simulink library "DYN_SRP"  (Simulink 8.8)
settings: Solver=ode45  StartTime=0.0  StopTime=10.0  RelTol=1e-3  EnableMultiTasking=on
undefined symbols (not defined in the file): CONSTANTS_par, DYN_SC_par
libraries: LIB_ROT x3, LIB_DYN x1, LIB_ENV x1
settings Model: Creator=alger  LastModifiedBy=alger

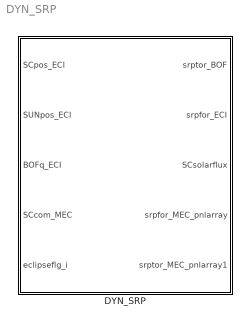
== system DYN_SRP ==
  DYN_SRP : Subsystem

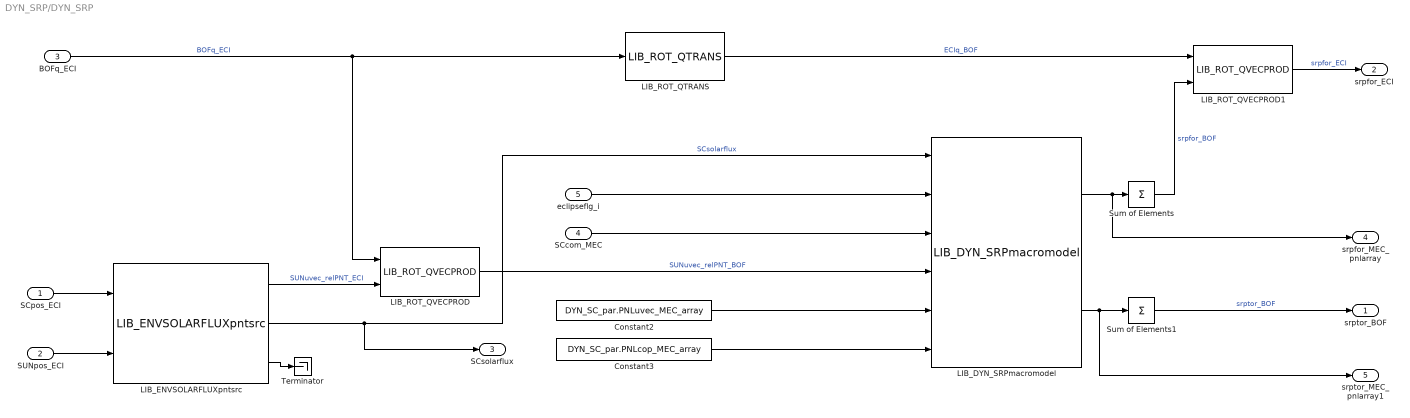
== system DYN_SRP/DYN_SRP ==
  SCpos_ECI : Inport  PortDimensions=3
  SUNpos_ECI : Inport  Port=2  PortDimensions=3
  BOFq_ECI : Inport  Port=3  PortDimensions=4  LockScale=on
  SCcom_MEC : Inport  Port=4  PortDimensions=3
  eclipseflg_i : Inport  Port=5  PortDimensions=1
  Constant2 : Constant  Value=DYN_SC_par.PNLuvec_MEC_array
  Constant3 : Constant  Value=DYN_SC_par.PNLcop_MEC_array
  LIB_DYN_SRPmacromodel : LIB_DYN/LIB_DYN_SRPmacromodel  N=DYN_SC_par.num_panels  C=CONSTANTS_par.C  pnlarea_array=DYN_SC_par.PNLarea_array  pnlcrd_array=DYN_SC_par.PNLcrdiffuse_array  pnlcrs_array=DYN_SC_par.PNLcrspecular_array
  LIB_ENVSOLARFLUXpntsrc : LIB_ENV/LIB_ENVSOLARFLUXpntsrc  solar_flux_ref=1367  solar_dist_ref=149597870700.0  zero_tol=695700000*5
  LIB_ROT_QTRANS : LIB_ROT/LIB_ROT_QTRANS
  LIB_ROT_QVECPROD : LIB_ROT/LIB_ROT_QVECPROD
  LIB_ROT_QVECPROD1 : LIB_ROT/LIB_ROT_QVECPROD
  Sum of Elements : Sum  Inputs=+  CollapseMode=Specified dimension  CollapseDim=2
  Sum of Elements1 : Sum  Inputs=+  CollapseMode=Specified dimension  CollapseDim=2
  Terminator : Terminator
  srptor_BOF : Outport  PortDimensions=3
  srpfor_ECI : Outport  Port=2  PortDimensions=3
  SCsolarflux : Outport  Port=3
  srpfor_MEC_pnlarray : Outport  Port=4
  srptor_MEC_pnlarray1 : Outport  Port=5
  wires:
  LIB_ROT_QVECPROD1/1 -> srpfor_ECI/1  "srpfor_ECI"
  Sum of Elements1/1 -> srptor_BOF/1  "srptor_BOF"
  SUNpos_ECI/1 -> LIB_ENVSOLARFLUXpntsrc/2
  SCpos_ECI/1 -> LIB_ENVSOLARFLUXpntsrc/1
  Constant3/1 -> LIB_DYN_SRPmacromodel/6
  Constant2/1 -> LIB_DYN_SRPmacromodel/5
  LIB_ROT_QTRANS/1 -> LIB_ROT_QVECPROD1/1  "ECIq_BOF"
  BOFq_ECI/1 -> LIB_ROT_QTRANS/1, LIB_ROT_QVECPROD/1  "BOFq_ECI"
  LIB_ROT_QVECPROD/1 -> LIB_DYN_SRPmacromodel/4  "SUNuvec_relPNT_BOF"
  LIB_ENVSOLARFLUXpntsrc/3 -> Terminator/1
  LIB_ENVSOLARFLUXpntsrc/1 -> LIB_ROT_QVECPROD/2  "SUNuvec_relPNT_ECI"
  LIB_ENVSOLARFLUXpntsrc/2 -> SCsolarflux/1, LIB_DYN_SRPmacromodel/1  "SCsolarflux"
  Sum of Elements/1 -> LIB_ROT_QVECPROD1/2  "srpfor_BOF"
  SCcom_MEC/1 -> LIB_DYN_SRPmacromodel/3
  eclipseflg_i/1 -> LIB_DYN_SRPmacromodel/2
  LIB_DYN_SRPmacromodel/1 -> srpfor_MEC_pnlarray/1, Sum of Elements/1
  LIB_DYN_SRPmacromodel/2 -> srptor_MEC_pnlarray1/1, Sum of Elements1/1
